simulink model "ConvFlow_markus"  (Simulink 6.2)
settings: Solver=FixedStepDiscrete  StartTime=0.0  StopTime=inf  FixedStep=.01  RelTol=1e-3
libraries: xpclib x1
settings Model: LastModifiedBy=mhauschild  ExtModeArmWhenConnect=off  BufferReuse=off
settings ConfigSet: SimulationMode=external
settings OptimizationCC: BlockReduction=off  OptimizeBlockIOStorage=off  BufferReuse=off  ExpressionFolding=off  LocalBlockOutputs=off
settings DebuggingCC: SolverPrmCheckMsg=warning
settings RTWCC: SystemTargetFile=xpctarget.tlc  TemplateMakefile=xpc_default_tmf  Description=xPC Target  ProcessScript=xpctarget_make_rtw_hook
settings xpcTargetCC: TargetFcnLib=ansi_tfl_tmw.mat  GenFloatMathFcnCalls=ANSI_C

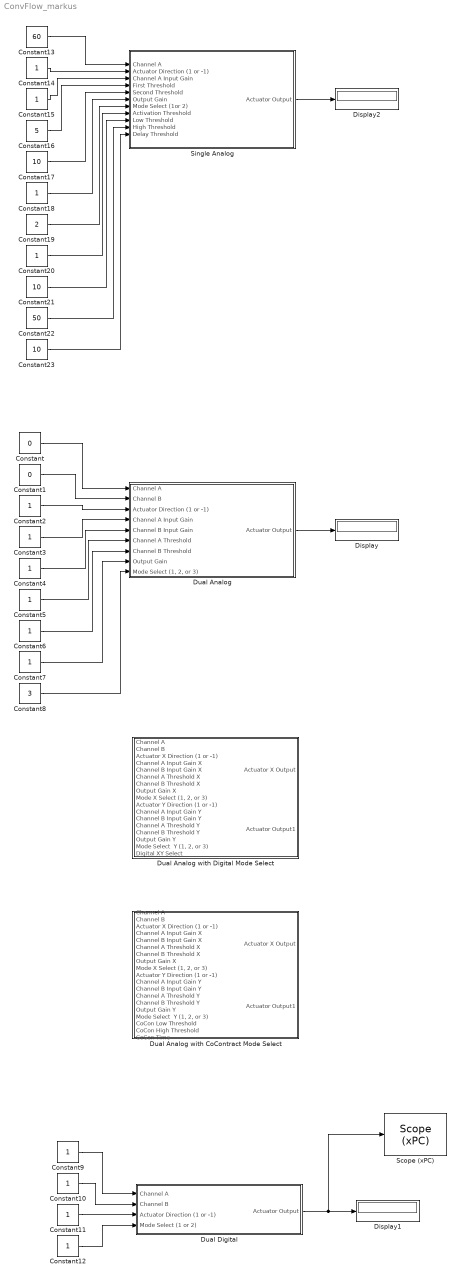
== system ConvFlow_markus ==
  Constant : Constant  Value=0
  Constant1 : Constant  Value=0
  Constant{2..7,9..12,14..15,18,20} (14 alike) : Constant
  Constant13 : Constant  Value=60
  Constant16 : Constant  Value=5
  Constant17 : Constant  Value=10
  Constant19 : Constant  Value=2
  Constant21 : Constant  Value=10
  Constant22 : Constant  Value=50
  Constant23 : Constant  Value=10
  Constant8 : Constant  Value=3
  Display : Display
  Display1 : Display
  Display2 : Display
  Dual Analog : Subsystem
  Dual Analog with CoContract Mode Select : Subsystem
  Dual Analog with Digital Mode Select : Subsystem
  Dual Digital : Subsystem
  "Scope (xPC) " : xpclib/Misc./Scope (xPC)   scopeno=1  scopetype=Target  autostart=on  viewmode=Numerical  formatstr='%15.6f'  grid=on  ylimits=[0,0]  nosamples=3  noprepostsamples=0  interleave=1  triggermode=FreeRun  triggersignal=1  triggerlevel=0.0  triggerslope=Either  triggerscope=1  triggersample=0  filename=data.dat  mode=Lazy  writesize=512  autorestart=off
  Single Analog : Subsystem
  wires:
  Dual Analog/1(Actuator Output) -> Display/1
  Constant/1 -> Dual Analog/1(Channel A)
  Constant1/1 -> Dual Analog/2(Channel B)
  Constant2/1 -> Dual Analog/3(Actuator Direction (1 or -1))
  Constant3/1 -> Dual Analog/4(Channel A Input Gain)
  Constant4/1 -> Dual Analog/5(Channel B Input Gain)
  Constant5/1 -> Dual Analog/6(Channel A Threshold)
  Constant6/1 -> Dual Analog/7(Channel B Threshold)
  Constant7/1 -> Dual Analog/8(Output Gain)
  Constant8/1 -> Dual Analog/9("Mode Select (1, 2, or 3)")
  Dual Digital/1(Actuator Output) -> Display1/1, "Scope (xPC) "/1
  Constant9/1 -> Dual Digital/1(Channel A)
  Constant10/1 -> Dual Digital/2(Channel B)
  Constant11/1 -> Dual Digital/3(Actuator Direction (1 or -1))
  Constant12/1 -> Dual Digital/4(Mode Select (1 or 2))
  Constant13/1 -> Single Analog/1(Channel A)
  Constant14/1 -> Single Analog/2(Actuator Direction (1 or -1))
  Constant15/1 -> Single Analog/3(Channel A Input Gain)
  Constant16/1 -> Single Analog/4(First Threshold)
  Constant17/1 -> Single Analog/5(Second Threshold)
  Constant18/1 -> Single Analog/6(Output Gain)
  Constant19/1 -> Single Analog/7(Mode Select (1or 2))
  Single Analog/1(Actuator Output) -> Display2/1
  Constant20/1 -> Single Analog/8(Activation Threshold)
  Constant23/1 -> Single Analog/11(Delay Threshold)
  Constant22/1 -> Single Analog/10(High Threshold)
  Constant21/1 -> Single Analog/9(Low Threshold)

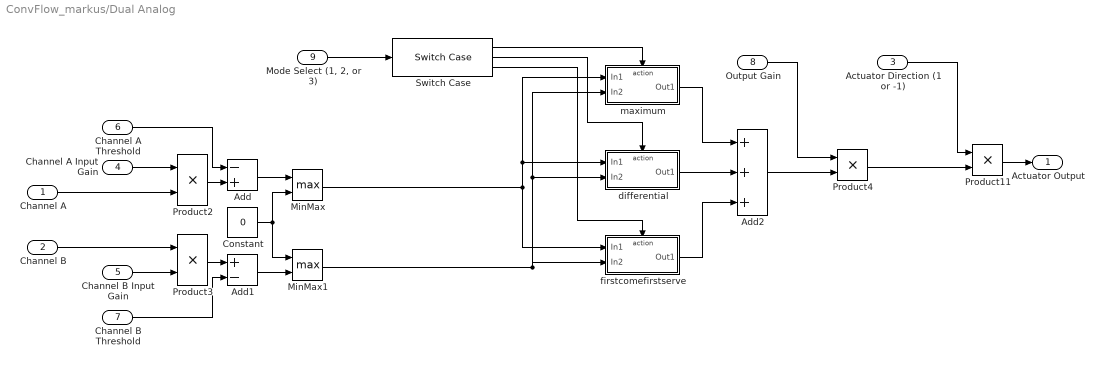
== system ConvFlow_markus/Dual Analog ==
  Channel A : Inport  Port=1  LatchInput=off
  Channel B : Inport  Port=2  LatchInput=off
  Actuator Direction (1 or -1) : Inport  Port=3  LatchInput=off
  Channel A Input Gain : Inport  Port=4  LatchInput=off
  Channel B Input Gain : Inport  Port=5  LatchInput=off
  Channel A Threshold : Inport  Port=6  LatchInput=off
  Channel B Threshold : Inport  Port=7  LatchInput=off
  Output Gain : Inport  Port=8  LatchInput=off
  "Mode Select (1, 2, or 3)" : Inport  Port=9  LatchInput=off
  Add : Sum  Inputs=-+  OutScaling=2^-10
  Add1 : Sum  Inputs=+-  OutScaling=2^-10
  Add2 : Sum  Inputs=+++  OutScaling=2^-10
  Constant : Constant  Value=0
  MinMax : MinMax  Function=max  Inputs=2
  MinMax1 : MinMax  Function=max  Inputs=2
  Product{2..4,11} (4 alike) : Product  RndMeth=Zero
  Switch Case : SwitchCase  CaseConditions={1, 2, 3}  CaseShowDefault=off
  differential : Subsystem  TreatAsAtomicUnit=on
  firstcomefirstserve : Subsystem  TreatAsAtomicUnit=on
  maximum : Subsystem  TreatAsAtomicUnit=on
  Actuator Output : Outport
  wires:
  Channel A/1 -> Product2/2
  Channel B/1 -> Product3/1
  Channel B Input Gain/1 -> Product3/2
  Channel A Input Gain/1 -> Product2/1
  Product3/1 -> Add1/1
  Product2/1 -> Add/2
  Channel B Threshold/1 -> Add1/2
  Channel A Threshold/1 -> Add/1
  Add/1 -> MinMax/1
  Add1/1 -> MinMax1/2
  Constant/1 -> MinMax/2, MinMax1/1
  Product4/1 -> Product11/2
  Product11/1 -> Actuator Output/1
  Actuator Direction (1 or -1)/1 -> Product11/1
  Switch Case/1 -> maximum/Action
  Switch Case/2 -> differential/Action
  Switch Case/3 -> firstcomefirstserve/Action
  "Mode Select (1, 2, or 3)"/1 -> Switch Case/1
  MinMax/1 -> maximum/1(In1), differential/1(In1), firstcomefirstserve/1(In1)
  MinMax1/1 -> maximum/2(In2), differential/2(In2), firstcomefirstserve/2(In2)
  maximum/1(Out1) -> Add2/1
  differential/1(Out1) -> Add2/2
  firstcomefirstserve/1(Out1) -> Add2/3
  Output Gain/1 -> Product4/1
  Add2/1 -> Product4/2

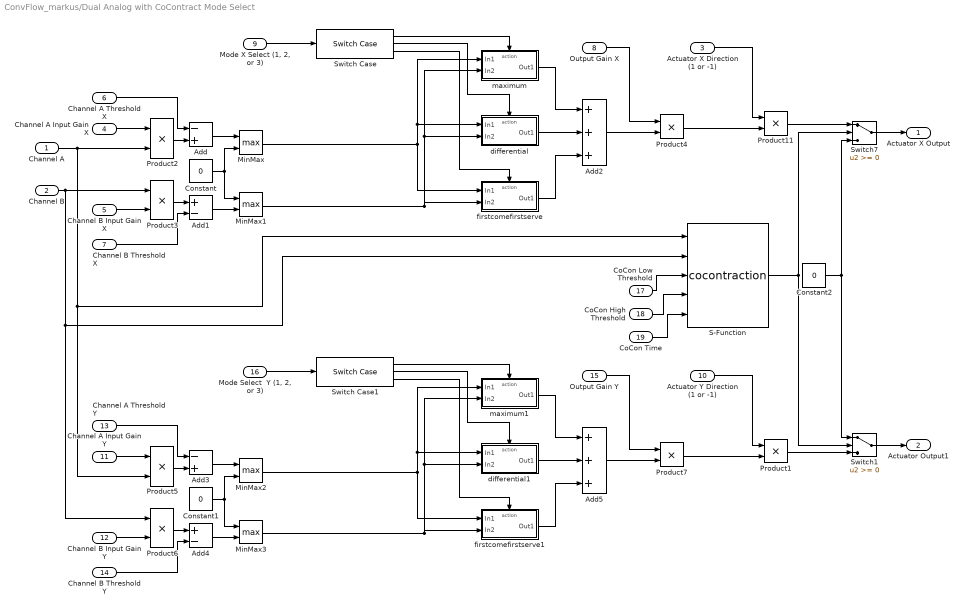
== system ConvFlow_markus/Dual Analog with CoContract Mode Select ==
  Channel A : Inport  Port=1  LatchInput=off
  Channel B : Inport  Port=2  LatchInput=off
  Actuator X Direction (1 or -1) : Inport  Port=3  LatchInput=off
  Channel A Input Gain X : Inport  Port=4  LatchInput=off
  Channel B Input Gain X : Inport  Port=5  LatchInput=off
  Channel A Threshold X : Inport  Port=6  LatchInput=off
  Channel B Threshold X : Inport  Port=7  LatchInput=off
  Output Gain X : Inport  Port=8  LatchInput=off
  "Mode X Select (1, 2, or 3)" : Inport  Port=9  LatchInput=off
  Actuator Y Direction (1 or -1) : Inport  Port=10  LatchInput=off
  Channel A Input Gain Y : Inport  Port=11  LatchInput=off
  Channel B Input Gain Y : Inport  Port=12  LatchInput=off
  Channel A Threshold Y : Inport  Port=13  LatchInput=off
  Channel B Threshold Y : Inport  Port=14  LatchInput=off
  Output Gain Y : Inport  Port=15  LatchInput=off
  "Mode Select  Y (1, 2, or 3)" : Inport  Port=16  LatchInput=off
  CoCon Low Threshold : Inport  Port=17  LatchInput=off
  CoCon High Threshold : Inport  Port=18  LatchInput=off
  CoCon Time : Inport  Port=19  LatchInput=off
  Add : Sum  Inputs=-+  OutScaling=2^-10
  Add1 : Sum  Inputs=+-  OutScaling=2^-10
  Add2 : Sum  Inputs=+++  OutScaling=2^-10
  Add3 : Sum  Inputs=-+  OutScaling=2^-10
  Add4 : Sum  Inputs=+-  OutScaling=2^-10
  Add5 : Sum  Inputs=+++  OutScaling=2^-10
  Constant : Constant  Value=0
  Constant1 : Constant  Value=0
  Constant2 : Constant  Value=0
  MinMax{,1..3} (4 alike) : MinMax  Function=max  Inputs=2
  Product{1..7,11} (8 alike) : Product  RndMeth=Zero
  S-Function : S-Function  FunctionName=cocontraction
  Switch Case : SwitchCase  CaseConditions={1, 2, 3}  CaseShowDefault=off
  Switch Case1 : SwitchCase  CaseConditions={1, 2, 3}  CaseShowDefault=off
  Switch1 : Switch
  Switch7 : Switch
  differential : Subsystem  TreatAsAtomicUnit=on
  differential1 : Subsystem  TreatAsAtomicUnit=on
  firstcomefirstserve : Subsystem  TreatAsAtomicUnit=on
  firstcomefirstserve1 : Subsystem  TreatAsAtomicUnit=on
  maximum : Subsystem  TreatAsAtomicUnit=on
  maximum1 : Subsystem  TreatAsAtomicUnit=on
  Actuator X Output : Outport
  Actuator Output1 : Outport  Port=2
  wires:
  Channel A/1 -> Product2/2, Product5/2, S-Function/1
  Channel B/1 -> Product3/1, Product6/1, S-Function/2
  Channel B Input Gain X/1 -> Product3/2
  Channel A Input Gain X/1 -> Product2/1
  Product3/1 -> Add1/1
  Product2/1 -> Add/2
  Channel B Threshold X/1 -> Add1/2
  Channel A Threshold X/1 -> Add/1
  Add/1 -> MinMax/1
  Add1/1 -> MinMax1/2
  Constant/1 -> MinMax/2, MinMax1/1
  Product4/1 -> Product11/2
  Actuator X Direction (1 or -1)/1 -> Product11/1
  Switch Case/1 -> maximum/Action
  Switch Case/2 -> differential/Action
  Switch Case/3 -> firstcomefirstserve/Action
  "Mode X Select (1, 2, or 3)"/1 -> Switch Case/1
  MinMax/1 -> maximum/1(In1), differential/1(In1), firstcomefirstserve/1(In1)
  MinMax1/1 -> maximum/2(In2), differential/2(In2), firstcomefirstserve/2(In2)
  maximum/1(Out1) -> Add2/1
  differential/1(Out1) -> Add2/2
  firstcomefirstserve/1(Out1) -> Add2/3
  Output Gain X/1 -> Product4/1
  Add2/1 -> Product4/2
  Channel B Input Gain Y/1 -> Product6/2
  Channel A Input Gain Y/1 -> Product5/1
  Product6/1 -> Add4/1
  Product5/1 -> Add3/2
  Channel B Threshold Y/1 -> Add4/2
  Channel A Threshold Y/1 -> Add3/1
  Add3/1 -> MinMax2/1
  Add4/1 -> MinMax3/2
  Constant1/1 -> MinMax2/2, MinMax3/1
  Product7/1 -> Product1/2
  Actuator Y Direction (1 or -1)/1 -> Product1/1
  Switch Case1/1 -> maximum1/Action
  Switch Case1/2 -> differential1/Action
  Switch Case1/3 -> firstcomefirstserve1/Action
  "Mode Select  Y (1, 2, or 3)"/1 -> Switch Case1/1
  MinMax2/1 -> maximum1/1(In1), differential1/1(In1), firstcomefirstserve1/1(In1)
  MinMax3/1 -> maximum1/2(In2), differential1/2(In2), firstcomefirstserve1/2(In2)
  maximum1/1(Out1) -> Add5/1
  differential1/1(Out1) -> Add5/2
  firstcomefirstserve1/1(Out1) -> Add5/3
  Output Gain Y/1 -> Product7/1
  Add5/1 -> Product7/2
  Switch7/1 -> Actuator X Output/1
  Switch1/1 -> Actuator Output1/1
  Product1/1 -> Switch1/3
  Product11/1 -> Switch7/1
  Constant2/1 -> Switch7/3, Switch1/1
  CoCon High Threshold/1 -> S-Function/4
  CoCon Time/1 -> S-Function/5
  S-Function/1 -> Switch7/2, Switch1/2
  CoCon Low Threshold/1 -> S-Function/3

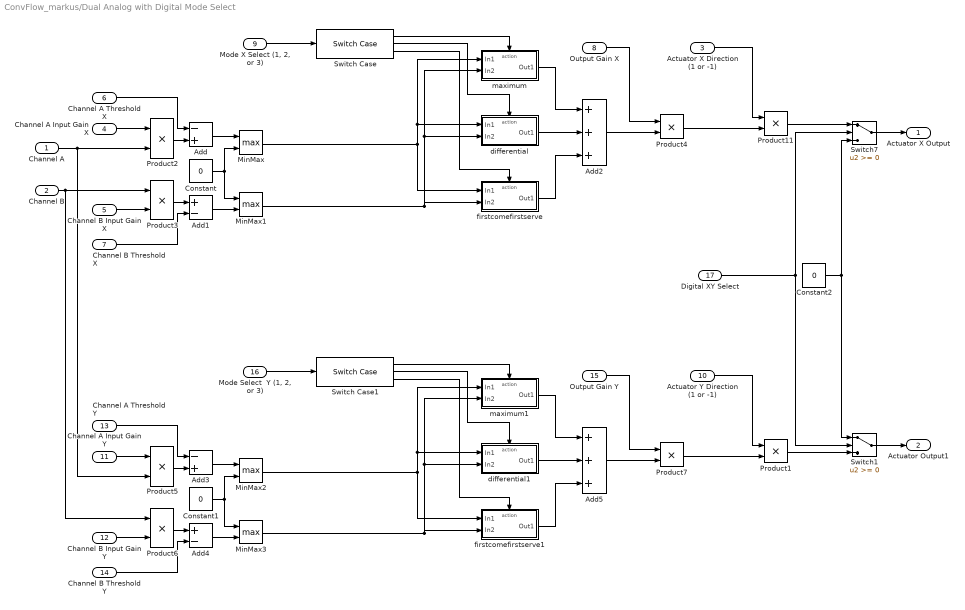
== system ConvFlow_markus/Dual Analog with Digital Mode Select ==
  Channel A : Inport  Port=1  LatchInput=off
  Channel B : Inport  Port=2  LatchInput=off
  Actuator X Direction (1 or -1) : Inport  Port=3  LatchInput=off
  Channel A Input Gain X : Inport  Port=4  LatchInput=off
  Channel B Input Gain X : Inport  Port=5  LatchInput=off
  Channel A Threshold X : Inport  Port=6  LatchInput=off
  Channel B Threshold X : Inport  Port=7  LatchInput=off
  Output Gain X : Inport  Port=8  LatchInput=off
  "Mode X Select (1, 2, or 3)" : Inport  Port=9  LatchInput=off
  Actuator Y Direction (1 or -1) : Inport  Port=10  LatchInput=off
  Channel A Input Gain Y : Inport  Port=11  LatchInput=off
  Channel B Input Gain Y : Inport  Port=12  LatchInput=off
  Channel A Threshold Y : Inport  Port=13  LatchInput=off
  Channel B Threshold Y : Inport  Port=14  LatchInput=off
  Output Gain Y : Inport  Port=15  LatchInput=off
  "Mode Select  Y (1, 2, or 3)" : Inport  Port=16  LatchInput=off
  Digital XY Select : Inport  Port=17  LatchInput=off
  Add : Sum  Inputs=-+  OutScaling=2^-10
  Add1 : Sum  Inputs=+-  OutScaling=2^-10
  Add2 : Sum  Inputs=+++  OutScaling=2^-10
  Add3 : Sum  Inputs=-+  OutScaling=2^-10
  Add4 : Sum  Inputs=+-  OutScaling=2^-10
  Add5 : Sum  Inputs=+++  OutScaling=2^-10
  Constant : Constant  Value=0
  Constant1 : Constant  Value=0
  Constant2 : Constant  Value=0
  MinMax{,1..3} (4 alike) : MinMax  Function=max  Inputs=2
  Product{1..7,11} (8 alike) : Product  RndMeth=Zero
  Switch Case : SwitchCase  CaseConditions={1, 2, 3}  CaseShowDefault=off
  Switch Case1 : SwitchCase  CaseConditions={1, 2, 3}  CaseShowDefault=off
  Switch1 : Switch
  Switch7 : Switch
  differential : Subsystem  TreatAsAtomicUnit=on
  differential1 : Subsystem  TreatAsAtomicUnit=on
  firstcomefirstserve : Subsystem  TreatAsAtomicUnit=on
  firstcomefirstserve1 : Subsystem  TreatAsAtomicUnit=on
  maximum : Subsystem  TreatAsAtomicUnit=on
  maximum1 : Subsystem  TreatAsAtomicUnit=on
  Actuator X Output : Outport
  Actuator Output1 : Outport  Port=2
  wires:
  Channel A/1 -> Product2/2, Product5/2
  Channel B/1 -> Product3/1, Product6/1
  Channel B Input Gain X/1 -> Product3/2
  Channel A Input Gain X/1 -> Product2/1
  Product3/1 -> Add1/1
  Product2/1 -> Add/2
  Channel B Threshold X/1 -> Add1/2
  Channel A Threshold X/1 -> Add/1
  Add/1 -> MinMax/1
  Add1/1 -> MinMax1/2
  Constant/1 -> MinMax/2, MinMax1/1
  Product4/1 -> Product11/2
  Actuator X Direction (1 or -1)/1 -> Product11/1
  Switch Case/1 -> maximum/Action
  Switch Case/2 -> differential/Action
  Switch Case/3 -> firstcomefirstserve/Action
  "Mode X Select (1, 2, or 3)"/1 -> Switch Case/1
  MinMax/1 -> maximum/1(In1), differential/1(In1), firstcomefirstserve/1(In1)
  MinMax1/1 -> maximum/2(In2), differential/2(In2), firstcomefirstserve/2(In2)
  maximum/1(Out1) -> Add2/1
  differential/1(Out1) -> Add2/2
  firstcomefirstserve/1(Out1) -> Add2/3
  Output Gain X/1 -> Product4/1
  Add2/1 -> Product4/2
  Channel B Input Gain Y/1 -> Product6/2
  Channel A Input Gain Y/1 -> Product5/1
  Product6/1 -> Add4/1
  Product5/1 -> Add3/2
  Channel B Threshold Y/1 -> Add4/2
  Channel A Threshold Y/1 -> Add3/1
  Add3/1 -> MinMax2/1
  Add4/1 -> MinMax3/2
  Constant1/1 -> MinMax2/2, MinMax3/1
  Product7/1 -> Product1/2
  Actuator Y Direction (1 or -1)/1 -> Product1/1
  Switch Case1/1 -> maximum1/Action
  Switch Case1/2 -> differential1/Action
  Switch Case1/3 -> firstcomefirstserve1/Action
  "Mode Select  Y (1, 2, or 3)"/1 -> Switch Case1/1
  MinMax2/1 -> maximum1/1(In1), differential1/1(In1), firstcomefirstserve1/1(In1)
  MinMax3/1 -> maximum1/2(In2), differential1/2(In2), firstcomefirstserve1/2(In2)
  maximum1/1(Out1) -> Add5/1
  differential1/1(Out1) -> Add5/2
  firstcomefirstserve1/1(Out1) -> Add5/3
  Output Gain Y/1 -> Product7/1
  Add5/1 -> Product7/2
  Switch7/1 -> Actuator X Output/1
  Switch1/1 -> Actuator Output1/1
  Product1/1 -> Switch1/3
  Product11/1 -> Switch7/1
  Digital XY Select/1 -> Switch7/2, Switch1/2
  Constant2/1 -> Switch7/3, Switch1/1

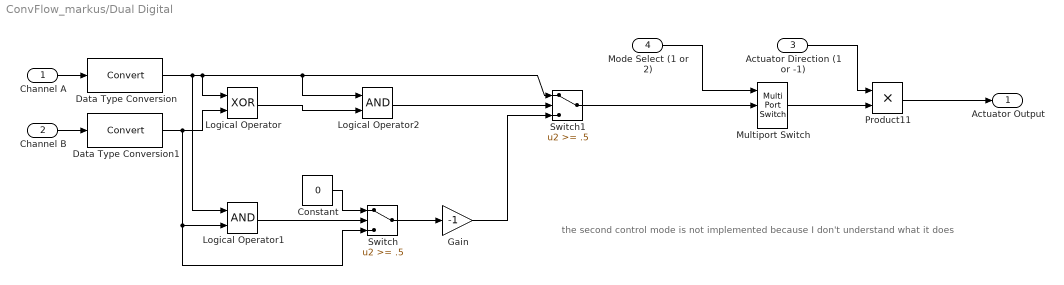
== system ConvFlow_markus/Dual Digital ==
  note: the second control mode is not implemented because I don't understand what it does
  Channel A : Inport  Port=1  LatchInput=off
  Channel B : Inport  Port=2  LatchInput=off
  Actuator Direction (1 or -1) : Inport  Port=3  LatchInput=off
  Mode Select (1 or 2) : Inport  Port=4  LatchInput=off
  Constant : Constant  Value=0
  Data Type Conversion : DataTypeConversion
  Data Type Conversion1 : DataTypeConversion
  Gain : Gain  Gain=-1
  Logical Operator : Logic  Operator=XOR  AllPortsSameDT=off  OutDataTypeMode=Boolean
  Logical Operator1 : Logic  AllPortsSameDT=off  OutDataTypeMode=Boolean
  Logical Operator2 : Logic  AllPortsSameDT=off  OutDataTypeMode=Boolean
  Multiport Switch : MultiPortSwitch  Inputs=2
  Product11 : Product  RndMeth=Zero
  Switch : Switch  Threshold=.5
  Switch1 : Switch  Threshold=.5
  Actuator Output : Outport
  wires:
  Channel A/1 -> Data Type Conversion/1
  Channel B/1 -> Data Type Conversion1/1
  Data Type Conversion/1 -> Logical Operator1/1, Logical Operator/1, Switch1/1, Logical Operator2/1
  Data Type Conversion1/1 -> Logical Operator/2, Logical Operator1/2, Switch/3
  Constant/1 -> Switch/1
  Logical Operator1/1 -> Switch/2
  Switch/1 -> Gain/1
  Gain/1 -> Switch1/3
  Actuator Direction (1 or -1)/1 -> Product11/1
  Mode Select (1 or 2)/1 -> Multiport Switch/1
  Switch1/1 -> Multiport Switch/2
  Multiport Switch/1 -> Product11/2
  Product11/1 -> Actuator Output/1
  Logical Operator2/1 -> Switch1/2
  Logical Operator/1 -> Logical Operator2/2

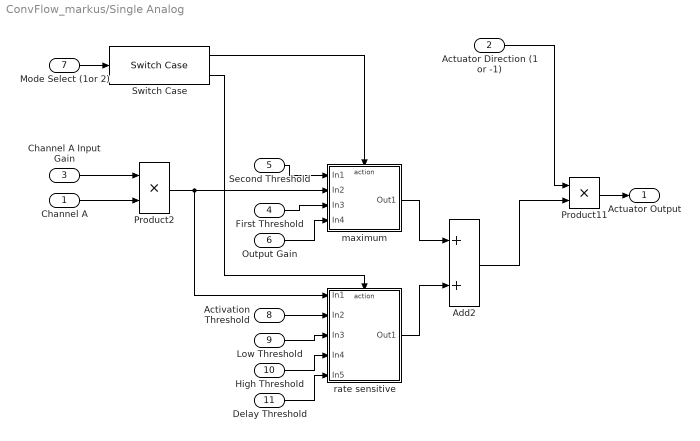
== system ConvFlow_markus/Single Analog ==
  Channel A : Inport  Port=1  LatchInput=off
  Actuator Direction (1 or -1) : Inport  Port=2  LatchInput=off
  Channel A Input Gain : Inport  Port=3  LatchInput=off
  First Threshold : Inport  Port=4  LatchInput=off
  Second Threshold : Inport  Port=5  LatchInput=off
  Output Gain : Inport  Port=6  LatchInput=off
  Mode Select (1or 2) : Inport  Port=7  LatchInput=off
  Activation Threshold : Inport  Port=8  LatchInput=off
  Low Threshold : Inport  Port=9  LatchInput=off
  High Threshold : Inport  Port=10  LatchInput=off
  Delay Threshold : Inport  Port=11  LatchInput=off
  Add2 : Sum  OutScaling=2^-10
  Product11 : Product  RndMeth=Zero
  Product2 : Product  RndMeth=Zero
  Switch Case : SwitchCase  CaseConditions={1, 2}  CaseShowDefault=off
  maximum : Subsystem  TreatAsAtomicUnit=on
  rate sensitive : Subsystem  TreatAsAtomicUnit=on
  Actuator Output : Outport
  wires:
  Product11/1 -> Actuator Output/1
  Actuator Direction (1 or -1)/1 -> Product11/1
  Channel A/1 -> Product2/2
  Channel A Input Gain/1 -> Product2/1
  Second Threshold/1 -> maximum/1(In1)
  Product2/1 -> maximum/2(In2), rate sensitive/1(In1)
  First Threshold/1 -> maximum/3(In3)
  Output Gain/1 -> maximum/4(In4)
  Activation Threshold/1 -> rate sensitive/2(In2)
  Low Threshold/1 -> rate sensitive/3(In3)
  High Threshold/1 -> rate sensitive/4(In4)
  Delay Threshold/1 -> rate sensitive/5(In5)
  Switch Case/1 -> maximum/Action
  Switch Case/2 -> rate sensitive/Action
  Mode Select (1or 2)/1 -> Switch Case/1
  maximum/1(Out1) -> Add2/1
  rate sensitive/1(Out1) -> Add2/2
  Add2/1 -> Product11/2

== system ConvFlow_markus/Dual Analog/differential ==
  In1 : Inport  Port=1  LatchInput=off
  In2 : Inport  Port=2  LatchInput=off
  Action Port : ActionPort  ActionType=case
  Subtract : Sum  Inputs=+-  OutScaling=2^-10
  Out1 : Outport  OutputWhenDisabled=reset  InitialOutput=[0]
  wires:
  In1/1 -> Subtract/1
  Subtract/1 -> Out1/1
  In2/1 -> Subtract/2

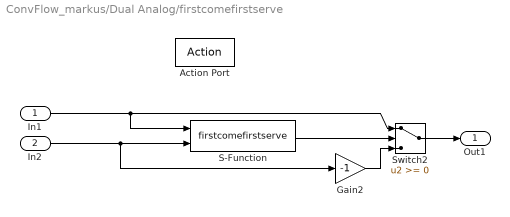
== system ConvFlow_markus/Dual Analog/firstcomefirstserve ==
  In1 : Inport  Port=1  LatchInput=off
  In2 : Inport  Port=2  LatchInput=off
  Action Port : ActionPort  ActionType=case
  Gain2 : Gain  Gain=-1
  S-Function : S-Function  FunctionName=firstcomefirstserve
  Switch2 : Switch
  Out1 : Outport  OutputWhenDisabled=reset  InitialOutput=[0]
  wires:
  Gain2/1 -> Switch2/3
  Switch2/1 -> Out1/1
  In1/1 -> S-Function/1, Switch2/1
  In2/1 -> S-Function/2, Gain2/1
  S-Function/1 -> Switch2/2

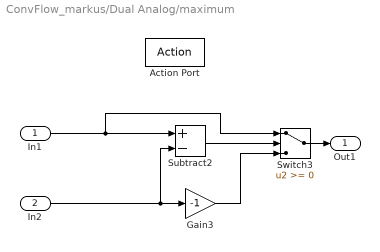
== system ConvFlow_markus/Dual Analog/maximum ==
  In1 : Inport  Port=1  LatchInput=off
  In2 : Inport  Port=2  LatchInput=off
  Action Port : ActionPort  ActionType=case
  Gain3 : Gain  Gain=-1
  Subtract2 : Sum  Inputs=+-  OutScaling=2^-10
  Switch3 : Switch
  Out1 : Outport  OutputWhenDisabled=reset  InitialOutput=[0]
  wires:
  In1/1 -> Subtract2/1, Switch3/1
  In2/1 -> Subtract2/2, Gain3/1
  Subtract2/1 -> Switch3/2
  Gain3/1 -> Switch3/3
  Switch3/1 -> Out1/1

== system ConvFlow_markus/Dual Analog with CoContract Mode Select/differential ==
  In1 : Inport  Port=1  LatchInput=off
  In2 : Inport  Port=2  LatchInput=off
  Action Port : ActionPort  ActionType=case
  Subtract : Sum  Inputs=+-  OutScaling=2^-10
  Out1 : Outport  OutputWhenDisabled=reset  InitialOutput=[0]
  wires:
  In1/1 -> Subtract/1
  Subtract/1 -> Out1/1
  In2/1 -> Subtract/2

== system ConvFlow_markus/Dual Analog with CoContract Mode Select/differential1 ==
  In1 : Inport  Port=1  LatchInput=off
  In2 : Inport  Port=2  LatchInput=off
  Action Port : ActionPort  ActionType=case
  Subtract : Sum  Inputs=+-  OutScaling=2^-10
  Out1 : Outport  OutputWhenDisabled=reset  InitialOutput=[0]
  wires:
  In1/1 -> Subtract/1
  Subtract/1 -> Out1/1
  In2/1 -> Subtract/2

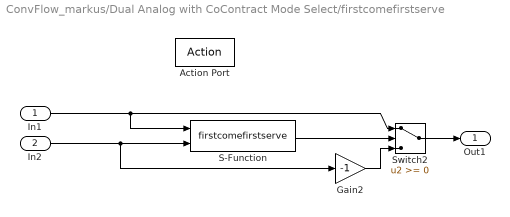
== system ConvFlow_markus/Dual Analog with CoContract Mode Select/firstcomefirstserve ==
  In1 : Inport  Port=1  LatchInput=off
  In2 : Inport  Port=2  LatchInput=off
  Action Port : ActionPort  ActionType=case
  Gain2 : Gain  Gain=-1
  S-Function : S-Function  FunctionName=firstcomefirstserve
  Switch2 : Switch
  Out1 : Outport  OutputWhenDisabled=reset  InitialOutput=[0]
  wires:
  Gain2/1 -> Switch2/3
  Switch2/1 -> Out1/1
  In1/1 -> S-Function/1, Switch2/1
  In2/1 -> S-Function/2, Gain2/1
  S-Function/1 -> Switch2/2

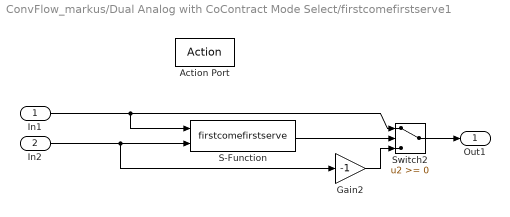
== system ConvFlow_markus/Dual Analog with CoContract Mode Select/firstcomefirstserve1 ==
  In1 : Inport  Port=1  LatchInput=off
  In2 : Inport  Port=2  LatchInput=off
  Action Port : ActionPort  ActionType=case
  Gain2 : Gain  Gain=-1
  S-Function : S-Function  FunctionName=firstcomefirstserve
  Switch2 : Switch
  Out1 : Outport  OutputWhenDisabled=reset  InitialOutput=[0]
  wires:
  Gain2/1 -> Switch2/3
  Switch2/1 -> Out1/1
  In1/1 -> S-Function/1, Switch2/1
  In2/1 -> S-Function/2, Gain2/1
  S-Function/1 -> Switch2/2

== system ConvFlow_markus/Dual Analog with CoContract Mode Select/maximum ==
  In1 : Inport  Port=1  LatchInput=off
  In2 : Inport  Port=2  LatchInput=off
  Action Port : ActionPort  ActionType=case
  Gain3 : Gain  Gain=-1
  Subtract2 : Sum  Inputs=+-  OutScaling=2^-10
  Switch3 : Switch
  Out1 : Outport  OutputWhenDisabled=reset  InitialOutput=[0]
  wires:
  In1/1 -> Subtract2/1, Switch3/1
  In2/1 -> Subtract2/2, Gain3/1
  Subtract2/1 -> Switch3/2
  Gain3/1 -> Switch3/3
  Switch3/1 -> Out1/1

== system ConvFlow_markus/Dual Analog with CoContract Mode Select/maximum1 ==
  In1 : Inport  Port=1  LatchInput=off
  In2 : Inport  Port=2  LatchInput=off
  Action Port : ActionPort  ActionType=case
  Gain3 : Gain  Gain=-1
  Subtract2 : Sum  Inputs=+-  OutScaling=2^-10
  Switch3 : Switch
  Out1 : Outport  OutputWhenDisabled=reset  InitialOutput=[0]
  wires:
  In1/1 -> Subtract2/1, Switch3/1
  In2/1 -> Subtract2/2, Gain3/1
  Subtract2/1 -> Switch3/2
  Gain3/1 -> Switch3/3
  Switch3/1 -> Out1/1

== system ConvFlow_markus/Dual Analog with Digital Mode Select/differential ==
  In1 : Inport  Port=1  LatchInput=off
  In2 : Inport  Port=2  LatchInput=off
  Action Port : ActionPort  ActionType=case
  Subtract : Sum  Inputs=+-  OutScaling=2^-10
  Out1 : Outport  OutputWhenDisabled=reset  InitialOutput=[0]
  wires:
  In1/1 -> Subtract/1
  Subtract/1 -> Out1/1
  In2/1 -> Subtract/2

== system ConvFlow_markus/Dual Analog with Digital Mode Select/differential1 ==
  In1 : Inport  Port=1  LatchInput=off
  In2 : Inport  Port=2  LatchInput=off
  Action Port : ActionPort  ActionType=case
  Subtract : Sum  Inputs=+-  OutScaling=2^-10
  Out1 : Outport  OutputWhenDisabled=reset  InitialOutput=[0]
  wires:
  In1/1 -> Subtract/1
  Subtract/1 -> Out1/1
  In2/1 -> Subtract/2

== system ConvFlow_markus/Dual Analog with Digital Mode Select/firstcomefirstserve ==
  In1 : Inport  Port=1  LatchInput=off
  In2 : Inport  Port=2  LatchInput=off
  Action Port : ActionPort  ActionType=case
  Gain2 : Gain  Gain=-1
  S-Function : S-Function  FunctionName=firstcomefirstserve
  Switch2 : Switch
  Out1 : Outport  OutputWhenDisabled=reset  InitialOutput=[0]
  wires:
  Gain2/1 -> Switch2/3
  Switch2/1 -> Out1/1
  In1/1 -> S-Function/1, Switch2/1
  In2/1 -> S-Function/2, Gain2/1
  S-Function/1 -> Switch2/2

== system ConvFlow_markus/Dual Analog with Digital Mode Select/firstcomefirstserve1 ==
  In1 : Inport  Port=1  LatchInput=off
  In2 : Inport  Port=2  LatchInput=off
  Action Port : ActionPort  ActionType=case
  Gain2 : Gain  Gain=-1
  S-Function : S-Function  FunctionName=firstcomefirstserve
  Switch2 : Switch
  Out1 : Outport  OutputWhenDisabled=reset  InitialOutput=[0]
  wires:
  Gain2/1 -> Switch2/3
  Switch2/1 -> Out1/1
  In1/1 -> S-Function/1, Switch2/1
  In2/1 -> S-Function/2, Gain2/1
  S-Function/1 -> Switch2/2

== system ConvFlow_markus/Dual Analog with Digital Mode Select/maximum ==
  In1 : Inport  Port=1  LatchInput=off
  In2 : Inport  Port=2  LatchInput=off
  Action Port : ActionPort  ActionType=case
  Gain3 : Gain  Gain=-1
  Subtract2 : Sum  Inputs=+-  OutScaling=2^-10
  Switch3 : Switch
  Out1 : Outport  OutputWhenDisabled=reset  InitialOutput=[0]
  wires:
  In1/1 -> Subtract2/1, Switch3/1
  In2/1 -> Subtract2/2, Gain3/1
  Subtract2/1 -> Switch3/2
  Gain3/1 -> Switch3/3
  Switch3/1 -> Out1/1

== system ConvFlow_markus/Dual Analog with Digital Mode Select/maximum1 ==
  In1 : Inport  Port=1  LatchInput=off
  In2 : Inport  Port=2  LatchInput=off
  Action Port : ActionPort  ActionType=case
  Gain3 : Gain  Gain=-1
  Subtract2 : Sum  Inputs=+-  OutScaling=2^-10
  Switch3 : Switch
  Out1 : Outport  OutputWhenDisabled=reset  InitialOutput=[0]
  wires:
  In1/1 -> Subtract2/1, Switch3/1
  In2/1 -> Subtract2/2, Gain3/1
  Subtract2/1 -> Switch3/2
  Gain3/1 -> Switch3/3
  Switch3/1 -> Out1/1

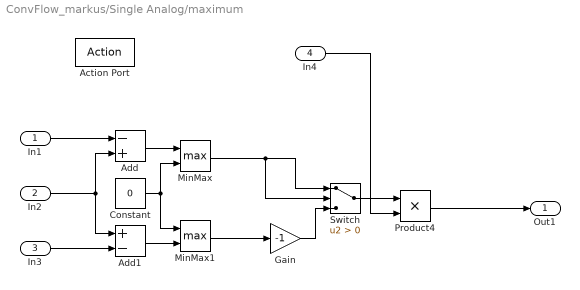
== system ConvFlow_markus/Single Analog/maximum ==
  In1 : Inport  Port=1  LatchInput=off
  In2 : Inport  Port=2  LatchInput=off
  In3 : Inport  Port=3  LatchInput=off
  In4 : Inport  Port=4  LatchInput=off
  Action Port : ActionPort  ActionType=case
  Add : Sum  Inputs=-+  OutScaling=2^-10
  Add1 : Sum  Inputs=+-  OutScaling=2^-10
  Constant : Constant  Value=0
  Gain : Gain  Gain=-1
  MinMax : MinMax  Function=max  Inputs=2
  MinMax1 : MinMax  Function=max  Inputs=2
  Product4 : Product  RndMeth=Zero
  Switch : Switch  Criteria=u2 > Threshold
  Out1 : Outport  OutputWhenDisabled=reset  InitialOutput=[0]
  wires:
  Gain/1 -> Switch/3
  Switch/1 -> Product4/1
  In4/1 -> Product4/2
  In3/1 -> Add1/2
  In1/1 -> Add/1
  Add/1 -> MinMax/1
  Add1/1 -> MinMax1/2
  Constant/1 -> MinMax/2, MinMax1/1
  MinMax/1 -> Switch/1, Switch/2
  MinMax1/1 -> Gain/1
  Product4/1 -> Out1/1
  In2/1 -> Add/2, Add1/1

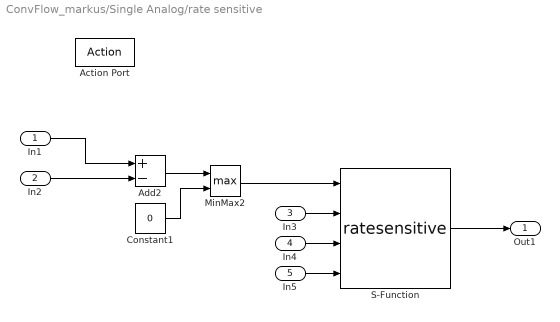
== system ConvFlow_markus/Single Analog/rate sensitive ==
  In1 : Inport  Port=1  LatchInput=off
  In2 : Inport  Port=2  LatchInput=off
  In3 : Inport  Port=3  LatchInput=off
  In4 : Inport  Port=4  LatchInput=off
  In5 : Inport  Port=5  LatchInput=off
  Action Port : ActionPort  ActionType=case
  Add2 : Sum  Inputs=+-  OutScaling=2^-10
  Constant1 : Constant  Value=0
  MinMax2 : MinMax  Function=max  Inputs=2
  S-Function : S-Function  FunctionName=ratesensitive
  Out1 : Outport  OutputWhenDisabled=reset  InitialOutput=[0]
  wires:
  Add2/1 -> MinMax2/1
  Constant1/1 -> MinMax2/2
  MinMax2/1 -> S-Function/1
  In3/1 -> S-Function/2
  In5/1 -> S-Function/4
  S-Function/1 -> Out1/1
  In1/1 -> Add2/1
  In2/1 -> Add2/2
  In4/1 -> S-Function/3
